simulink model "sy1_08022311"  (R2022b)
settings: Solver=VariableStepAuto  StartTime=0.0  StopTime=100  RelTol=1e-3
settings Model: Creator=赵晨琨  LastModifiedBy=ASUS
settings SolverCC: AlgebraicLoopSolver=TrustRegion
settings DataIOCC: Refine=3
settings DebuggingCC: UnconnectedInputMsg=warning  UnconnectedOutputMsg=warning  UnconnectedLineMsg=warning  SFMachineParentedDataDiag=warning
settings ModelReferenceCC: EnableRefExpFcnMdlSchedulingChecks=on

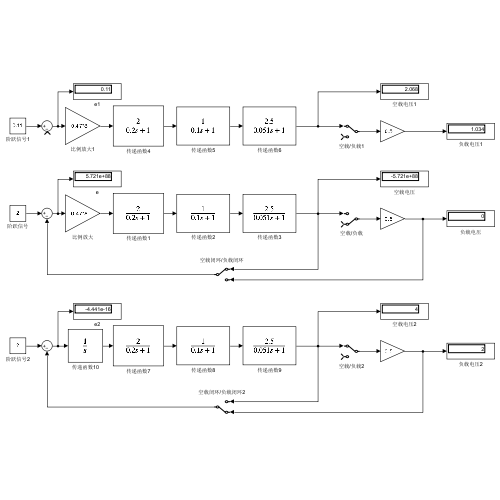
[thumbnail: Simulink's stored preview of the top-level diagram]
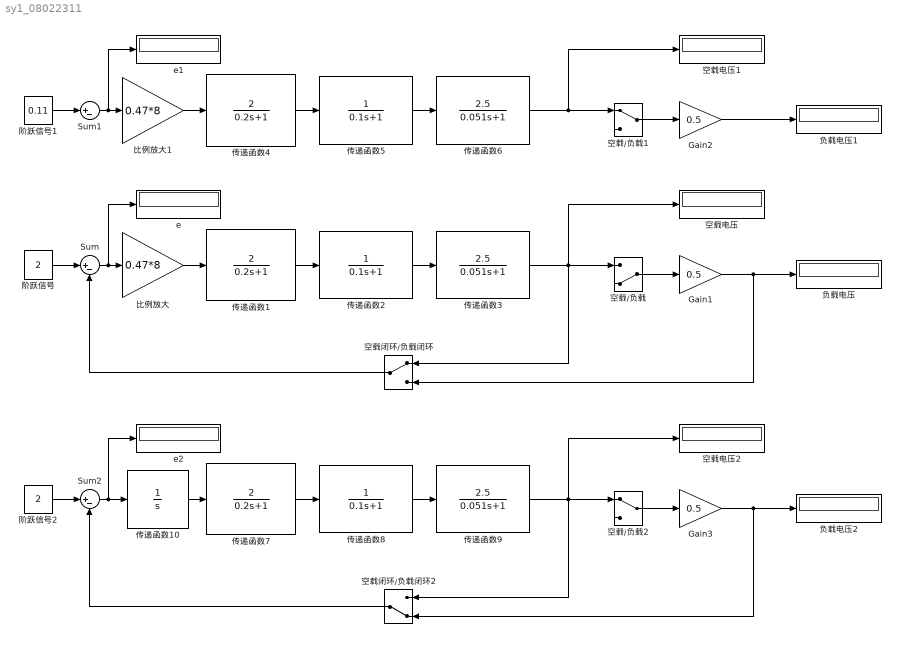
== system sy1_08022311 ==
  Gain1 : Gain  Gain=0.5
  Gain2 : Gain  Gain=0.5
  Gain3 : Gain  Gain=0.5
  Sum : Sum  Inputs=|+-
  Sum1 : Sum  Inputs=|+-
  Sum2 : Sum  Inputs=|+-
  e : Display
  e1 : Display
  e2 : Display
  传递函数1 : TransferFcn  Numerator=[2]  Denominator=[0.2 1]
  传递函数10 : TransferFcn  Denominator=[1 0]
  传递函数2 : TransferFcn  Denominator=[0.1 1]
  传递函数3 : TransferFcn  Numerator=[2.5]  Denominator=[0.051 1]
  传递函数4 : TransferFcn  Numerator=[2]  Denominator=[0.2 1]
  传递函数5 : TransferFcn  Denominator=[0.1 1]
  传递函数6 : TransferFcn  Numerator=[2.5]  Denominator=[0.051 1]
  传递函数7 : TransferFcn  Numerator=[2]  Denominator=[0.2 1]
  传递函数8 : TransferFcn  Denominator=[0.1 1]
  传递函数9 : TransferFcn  Numerator=[2.5]  Denominator=[0.051 1]
  比例放大 : Gain  Gain=0.47*8
  比例放大1 : Gain  Gain=0.47*8
  空载/负载 : ManualSwitch  CurrentSetting=0
  空载/负载1 : ManualSwitch
  空载/负载2 : ManualSwitch
  空载电压 : Display
  空载电压1 : Display
  空载电压2 : Display
  空载闭环/负载闭环 : ManualSwitch
  空载闭环/负载闭环2 : ManualSwitch  CurrentSetting=0
  负载电压 : Display
  负载电压1 : Display
  负载电压2 : Display
  阶跃信号 : Constant  Value=2
  阶跃信号1 : Constant  Value=0.11
  阶跃信号2 : Constant  Value=2
  wires:
  传递函数1/1 -> 传递函数2/1
  比例放大/1 -> 传递函数1/1
  传递函数2/1 -> 传递函数3/1
  传递函数3/1 -> 空载闭环/负载闭环/1, 空载电压/1, 空载/负载/1
  空载/负载/1 -> Gain1/1
  Gain1/1 -> 空载闭环/负载闭环/2, 负载电压/1
  阶跃信号/1 -> Sum/1
  Sum/1 -> e/1, 比例放大/1
  空载闭环/负载闭环/1 -> Sum/2
  Sum1/1 -> e1/1, 比例放大1/1
  Gain2/1 -> 负载电压1/1
  传递函数5/1 -> 传递函数6/1
  传递函数4/1 -> 传递函数5/1
  比例放大1/1 -> 传递函数4/1
  空载/负载1/1 -> Gain2/1
  传递函数6/1 -> 空载电压1/1, 空载/负载1/1
  阶跃信号1/1 -> Sum1/1
  Sum2/1 -> 传递函数10/1, e2/1
  Gain3/1 -> 空载闭环/负载闭环2/2, 负载电压2/1
  传递函数8/1 -> 传递函数9/1
  传递函数7/1 -> 传递函数8/1
  传递函数10/1 -> 传递函数7/1
  空载闭环/负载闭环2/1 -> Sum2/2
  空载/负载2/1 -> Gain3/1
  传递函数9/1 -> 空载闭环/负载闭环2/1, 空载电压2/1, 空载/负载2/1
  阶跃信号2/1 -> Sum2/1
